simulink model "reactor"  (R2016b)
settings: Solver=ode45  StartTime=0.0  StopTime=30  FixedStep=0.1  RelTol=1e-12  EnableMultiTasking=on
settings Model: Creator=amal029_old  LastModifiedBy=amal029_old
settings SolverCC: ZeroCrossAlgorithm=Adaptive  AutoInsertRateTranBlk=on
settings DataIOCC: LimitDataPoints=on
settings OptimizationCC: LifeSpan=inf
settings DebuggingCC: AllowSymbolicDim=off  SFUnexpectedBacktrackingDiag=warning  SFNoUnconditionalDefaultTransitionDiag=warning  SFExecutionAtInitializationDiag=none
settings GRTTargetCC: TargetLangStandard=C89/C90 (ANSI)
settings ConfigComp: CovMetricSettings=dw  CovHtmlReporting=on  CovSaveCumulativeToWorkspaceVar=on  CovSaveSingleToWorkspaceVar=on  CovShowResultsExplorer=off  CovExternalEMLEnable=off

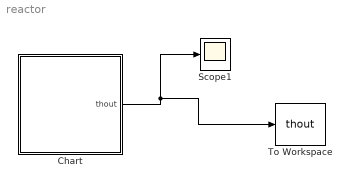
== system reactor ==
  Chart : Stateflow chart  TreatAsAtomicUnit=on
  Scope1 : Scope
  To Workspace : ToWorkspace  VariableName=thout  SampleTime=-1
      settings: Save2DSignal=2-D array (concatenate along first dimension)
  wires:
  Chart/1(thout) -> To Workspace/1, Scope1/1

== stateflow chart reactor/Chart ==
  settings: updateMethod=CONTINUOUS
  state State2
    du:
    x_dot=1.0; y_dot=1.0; th_dot=v1;thout=th;
  state State3
    du:
    x_dot=1.0; y_dot=1.0; th_dot=v2; thout=th;
  state State1
    du:
    x_dot=1.0; y_dot=1.0;
    th_dot=vr; thout=th;
  state State4
  State1 -> State2 [order 1] : [th >= thM && x >= T1]
  State2 -> State1 : [th <= thm]
  (default) -> State1 : {x=T1; y=T2; th=11.5; thout=th;}
  State1 -> State3 [order 2] : [th>=thM && y >= T2]
  State3 -> State1 : [th<=thm]
  State1 -> State4 [order 3] : [th >= thM && y < T2 && x < T1]
  data: x local; th local; y local; T1 constant double size=1 =10.0; T2 constant double size=1 =10.0; thM constant double size=1 =20.0; thm constant double size=1 =5; vr constant double size=1 =10.5; v1 constant double size=1 =-1.3; v2 constant double size=1 =-2.7; thout output
  data x settings: updateMethod=SF_CONTINUOUS_TIME_DATA
  data th settings: updateMethod=SF_CONTINUOUS_TIME_DATA
  data y settings: updateMethod=SF_CONTINUOUS_TIME_DATA
